simulink model "REI_circuit"  (R2021a)
settings: Solver=VariableStepAuto  StartTime=0.0  StopTime=20  RelTol=1e-3
values from neighbouring files (symbols this model uses):
  KLQR = KsLQR(:,1:4)    [REI.m]
libraries: cstblocks x5
settings Model: Creator=sofia  LastModifiedBy=sofia

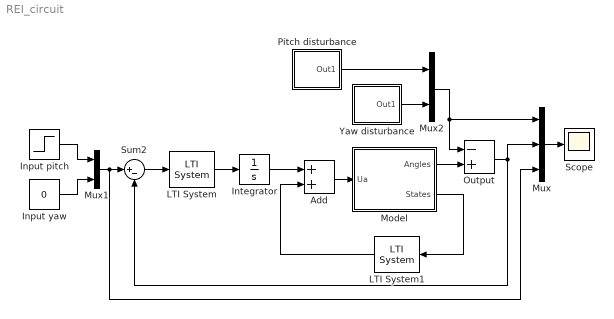
== system REI_circuit ==
  Add : Sum
  Input pitch : Step  After=0.583  SampleTime=0
  Input yaw : Constant  Value=0
  Integrator : Integrator
  LTI System : cstblocks/LTI System  sys=KiLQR  IC=[]
  LTI System1 : cstblocks/LTI System  sys=-KLQR  IC=[]
  Model : Subsystem
  Mux : Mux  Inputs=3
  Mux1 : Mux  Inputs=2
  Mux2 : Mux  Inputs=2
  Output : Sum  Inputs=-+
  Pitch disturbance : Subsystem
  Scope : Scope
  Sum2 : Sum  Inputs=|+-
  Yaw disturbance : Subsystem
  wires:
  Add/1 -> Model/1(Ua)
  Model/2(States) -> LTI System1/1
  Integrator/1 -> Add/1
  Mux/1 -> Scope/1
  Sum2/1 -> LTI System/1
  LTI System/1 -> Integrator/1
  LTI System1/1 -> Add/2
  Model/1(Angles) -> Output/2
  Output/1 -> Mux/2, Sum2/2
  Input pitch/1 -> Mux1/1
  Mux1/1 -> Mux/3, Sum2/1
  Input yaw/1 -> Mux1/2
  Pitch disturbance/1(Out1) -> Mux2/1
  Yaw disturbance/1(Out1) -> Mux2/2
  Mux2/1 -> Output/1, Mux/1

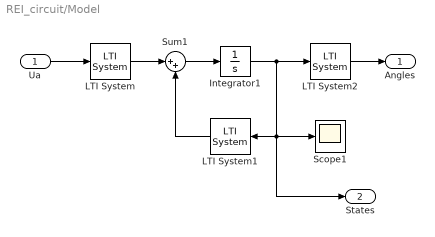
== system REI_circuit/Model ==
  Ua : Inport
  Integrator1 : Integrator
  LTI System : cstblocks/LTI System  sys=B  IC=[]
  LTI System1 : cstblocks/LTI System  sys=A  IC=[]
  LTI System2 : cstblocks/LTI System  sys=C  IC=[]
  Scope1 : Scope
  Sum1 : Sum  Inputs=|++
  Angles : Outport
  States : Outport  Port=2  PortDimensions=4
  wires:
  Ua/1 -> LTI System/1
  Sum1/1 -> Integrator1/1
  Integrator1/1 -> LTI System2/1, States/1, Scope1/1, LTI System1/1
  LTI System2/1 -> Angles/1
  LTI System1/1 -> Sum1/2
  LTI System/1 -> Sum1/1

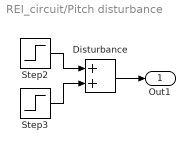
== system REI_circuit/Pitch disturbance ==
  Disturbance : Sum
  Step2 : Step  Time=13  After=0.2  SampleTime=1
  Step3 : Step  Time=15  After=-0.2  SampleTime=1
  Out1 : Outport
  wires:
  Step2/1 -> Disturbance/1
  Step3/1 -> Disturbance/2
  Disturbance/1 -> Out1/1

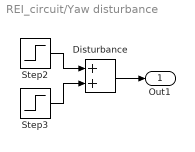
== system REI_circuit/Yaw disturbance ==
  Disturbance : Sum
  Step2 : Step  Time=10  After=0  SampleTime=1
  Step3 : Step  Time=12  After=0  SampleTime=1
  Out1 : Outport
  wires:
  Step2/1 -> Disturbance/1
  Step3/1 -> Disturbance/2
  Disturbance/1 -> Out1/1
